simulink model "Week2_Problem3"  (R2020a)
settings: Solver=VariableStepAuto  StartTime=0.0  StopTime=120  RelTol=1e-3
values from neighbouring files (symbols this model uses):
  b = 50.0    [ModelData.sldd]
  D = 1.0    [ModelData.sldd]
  I = 1.0    [ModelData.sldd]
  m = 1000.0    [ModelData.sldd]
  P = 1.0    [ModelData.sldd]
settings Model: DataDictionary=ModelData.sldd  Creator=tnradm  LastModifiedBy=tnradm

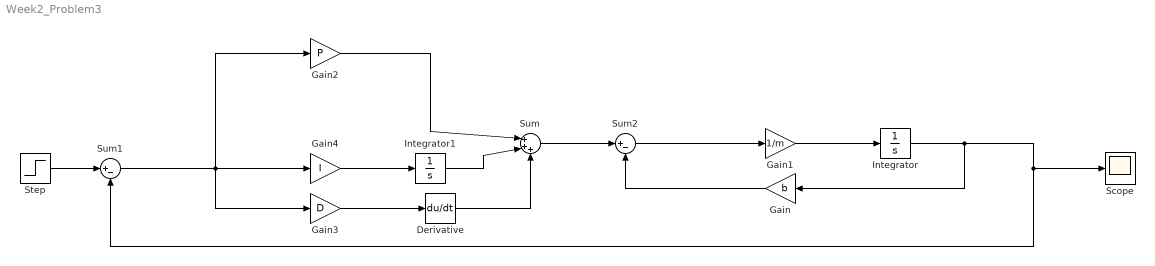
== system Week2_Problem3 ==
  " Scope " : Scope
  Derivative : Derivative
  Gain : Gain  Gain=b
  Gain1 : Gain  Gain=1/m
  Gain2 : Gain  Gain=P
  Gain3 : Gain  Gain=D
  Gain4 : Gain  Gain=I
  Integrator : Integrator
  Integrator1 : Integrator
  "Step " : Step  Time=0  After=u  SampleTime=0
  Sum : Sum  Inputs=|+++
  Sum1 : Sum  Inputs=|+-
  Sum2 : Sum  Inputs=|+-
  wires:
  "Step "/1 -> Sum1/1
  Integrator/1 -> Gain/1, " Scope "/1, Sum1/2
  Gain4/1 -> Integrator1/1
  Sum1/1 -> Gain2/1, Gain3/1, Gain4/1
  Gain2/1 -> Sum/1
  Integrator1/1 -> Sum/2
  Derivative/1 -> Sum/3
  Gain3/1 -> Derivative/1
  Sum/1 -> Sum2/1
  Sum2/1 -> Gain1/1
  Gain/1 -> Sum2/2
  Gain1/1 -> Integrator/1
